simulink model "regcontrol_model_3ph"  (R2018b)
settings: Solver=VariableStepAuto  StartTime=0.0  StopTime=10.0  RelTol=1e-3
values from neighbouring files (symbols this model uses):
  BandWidth = Simulink.Parameter    [start.m]
  BaseVoltage = Simulink.Parameter    [start.m]
  CogenEnabled = false    [regcontrol_emulator.m]    (also in start.m = Simulink.Parameter)
  ElementTerminal = 0    [start.m]
  FPTphase = Simulink.Parameter(FPTphases.DEFAULT)    [regcontrol_emulator.m]    (also in start.m = 1)
  InCogenMode = false    [regcontrol_emulator.m]
  InReverseMode = false    [regcontrol_emulator.m]
  IsReversible = Simulink.Parameter    [start.m]
  LastHandle = RecentExecuted(1,NewCtrlQueueFields.Handle, end)    [LogEvent_1ph.m]    (also in LogEvent_1ph_old.m)
  LDC_Z = Simulink.Parameter    [start.m]
  MaxTap = 1.10    (= 1.1)    [Transformer.m]
  MinTap = 0.90    (= 0.9)    [Transformer.m]
  PTratio = Simulink.Parameter    [start.m]
  R = 0    [start.m]
  RevBand = Simulink.Parameter    [start.m]
  RevVreg = Simulink.Parameter    [start.m]
  TapLimitPerChange = Simulink.Parameter    [start.m]
  UsingRegulatedBus = Simulink.Parameter    [start.m]
  Vlimit = Simulink.Parameter    [start.m]
  Vreg = Simulink.Parameter    [start.m]
  X = 0    [start.m]
undefined symbols (not defined in the file or in its folder): Armed, ControlledTransformerConnection, ControlledTransformerCurrents, ControlledTransformerPowers, ControlledTransformerVoltages, CTRating, DeltaDirection, IsInverseTime, LastQueue, LookingForward, m, n, NumConductors, NumPhases, PresentTap, RevBackHandle, RevDelay, ReversePending, RevHandle, revLDC_Z, RevPowerThreshold, revR, revX, TapDelay, TapIncrement, TapWinding, TimeDelay, TimeInSec, VTerminal
(part 4 of 4)

== stateflow chart regcontrol_model_3ph/Action Coordinator ==
  state ResendActions [parallel]
    settings: executionOrder=1
    state Asleep
      ex: IncrHandle;
      currHandle;
    note: Receive a push message
        |
        | Repackage message for the Queue, adding device index
        | Assign a handle and send it back to RegControl
        |
        | Send expanded push message to the Queue
    state Update2
      en:
      msgData = uint8(In2.data);
      deviceIndex = 2;
      if CodesIn(deviceIndex) == ...
      double(ActionCodes.ACTION_REVERSE)
      Handle2.data = currHandle;
      send(Handle2);
      end
    state Update1
      en:
      msgData = uint8(In1.data);
      deviceIndex = 1;
      if CodesIn(deviceIndex) == ...
      double(ActionCodes.ACTION_REVERSE)
      Handle1.data = currHandle;
      send(Handle1);
      end
    state Update3
      en:
      msgData = uint8(In3.data);
      deviceIndex = 3;
      if CodesIn(deviceIndex) == ...
      double(ActionCodes.ACTION_REVERSE)
      Handle3.data = currHandle;
      send(Handle3);
      end
    state SendUpdated
      en:
      Phases = Phases + 1;
      Out.data = [msgData; deviceIndex; currHandle];
      send(Out);
      send(CheckNumActions, DelaySolution);
    (default) -> ResendActions.Asleep
    SendUpdated -> ResendActions.Asleep
    ResendActions.Asleep -> Update1 [order 1] : In1
    ResendActions.Asleep -> Update2 [order 2] : In2
    ResendActions.Asleep -> Update3 [order 3] : In3
    Update3 -> SendUpdated
    Update1 -> SendUpdated
    Update2 -> SendUpdated
  state DelaySolution [parallel]
    settings: executionOrder=2
    state Asleep
    state ParseNumActions
      en: LocalNumActions = NumActions.data;
      discard(NumActions);
      length(NumActions);
    note: Example Behavior:
        | Receive NumActions message and store its value
        | Phases (# phases pushing/deleting from queue) < LocalNumActions
        | Because push/delete message is still in message queue
        | Receive CheckNumActions action
        | Because another phase's data has been processed
        | Phases == LocalNumActions
        | Send ActionsDone message to initiate Solution
    state SendActionsDone
      en: send(ActionsDone);
    (default) -> DelaySolution.Asleep
    (junction 50) -> DelaySolution.Asleep [order 2]
    DelaySolution.Asleep -> (junction 50) [order 2] : CheckNumActions
    DelaySolution.Asleep -> ParseNumActions [order 1] : NumActions
    ParseNumActions -> (junction 50)
    (junction 50) -> SendActionsDone [order 1] : [Phases == LocalNumActions]
  data: Handle1 output uint8 =uint8(0); Handle2 output uint8 =uint8(0); Handle3 output uint8 =uint8(0); In1 input Enum: QueueActions size=1; In2 input Enum: QueueActions size=1; In3 input Enum: QueueActions size=1; Out output uint8 size=3 =uint8([0;0;0]); msgData local uint8; deviceIndex local uint8; currHandle output uint8 =uint8(0); LastHandle input uint8; handleWriteFlag local boolean =false; CodesIn input double size=3; ActionsDone output boolean =true; NumActions input uint8; Phases local uint8 =uint8(0); LocalNumActions local uint8 =uint8(0)
  events: CheckNumActions local FUNCTION_CALL_EVENT
  function IncrHandle:
    | function IncrHandle
    |     if ~handleWriteFlag % resets to false on every simulation run
    |         currHandle = LastHandle;
    |         handleWriteFlag = true;
    |     end
    |     currHandle = currHandle + 1;
    | end

== stateflow chart regcontrol_model_3ph/SolverStarter ==
  state Asleep
  state IncrNumActions [function]
    (default) -> (junction 69) : {NumActions.data = NumActions.data + 1;
        | }
  state IncrPhasesDone
    en:
    PhasesDone = PhasesDone + 1;
  state WaitForActionsDone
    en: send(NumActions);
  state SendAllDone
    en: send(Out);
  (default) -> Asleep
  SendAllDone -> Asleep
  Asleep -> (junction 38) [order 1] : In1
  Asleep -> (junction 48) [order 3] : In2
  Asleep -> (junction 60) [order 2] : In3
  IncrPhasesDone -> Asleep [order 2]
  (junction 38) -> (junction 39) [order 1] : [In1.data == uint8(DoneMsg.QUEUE_ACTION)]
  (junction 60) -> (junction 56) [order 1] : [In3.data == uint8(DoneMsg.QUEUE_ACTION)]
  (junction 48) -> (junction 46) [order 1] : [In2.data == uint8(DoneMsg.QUEUE_ACTION)]
  (junction 38) -> (junction 40) [order 2]
  (junction 39) -> (junction 41) : {IncrNumActions;}
  (junction 60) -> (junction 57) [order 2]
  (junction 56) -> (junction 58) : {IncrNumActions;}
  (junction 48) -> (junction 51) [order 2]
  (junction 46) -> (junction 45) : {IncrNumActions;}
  (junction 41) -> (junction 40)
  (junction 58) -> (junction 57)
  (junction 45) -> (junction 51)
  (junction 40) -> IncrPhasesDone
  (junction 57) -> IncrPhasesDone
  (junction 51) -> IncrPhasesDone
  IncrPhasesDone -> WaitForActionsDone [order 1] : [PhasesDone == 3]
  WaitForActionsDone -> SendAllDone : ActionsDone
  data: NumActions output uint8 =uint8(0); ActionsDone input boolean; In1 input uint8 size=1; In2 input uint8 size=1; In3 input uint8 size=1; Out output boolean size=1 =true; PhasesDone local uint8 =uint8(0)

== stateflow chart regcontrol_model_3ph/DoPendingAction ==
  state Asleep
  state UpdateDevice
    en:
    msgData = In.data(1);
    deviceIndex = In.data(2);
    discard(In);
  state Send1
    en:
    Out1.data = msgData;
    send(Out1);
  state Send2
    en:
    Out2.data = msgData;
    send(Out2);
  state Send3
    en:
    Out3.data = msgData;
    send(Out3);
    send(PendingActionsCompleted);
  state SendPendingActionsCompleted
    en: send(PendingActionsCompleted);
  (default) -> Asleep
  (junction 48) -> Asleep [commented out]
  Asleep -> UpdateDevice : In
  (junction 44) -> UpdateDevice [commented out]
  UpdateDevice -> Send1 [order 1] : [deviceIndex == 1]
  UpdateDevice -> Send2 [order 2] : [deviceIndex == 2]
  UpdateDevice -> Send3 [order 3] : [deviceIndex == 3]
  Send1 -> (junction 26)
  Send2 -> (junction 26)
  Send3 -> (junction 26) : In3
  (junction 26) -> SendPendingActionsCompleted : {send(PendingActionsCompleted);}
  (junction 26) -> (junction 43) [commented out]
  (junction 43) -> (junction 44) [commented out] : [length(In) > 0]
  (junction 43) -> (junction 45) [commented out]
  (junction 45) -> (junction 48) [commented out]
  data: msgData local double; deviceIndex local double =double(0); In input double size=2; Out1 output double size=1 =0; Out2 output double size=1 =0; Out3 output double size=1 =0; In3 input boolean; PendingActionsCompleted output boolean =true
